simulink model "simu_hapstik_1"  (Simulink 7.7)
settings: Solver=ode45  StartTime=0.0  StopTime=25  RelTol=1e-3
settings Model: Creator=André Frank  LastModifiedBy=André Frank

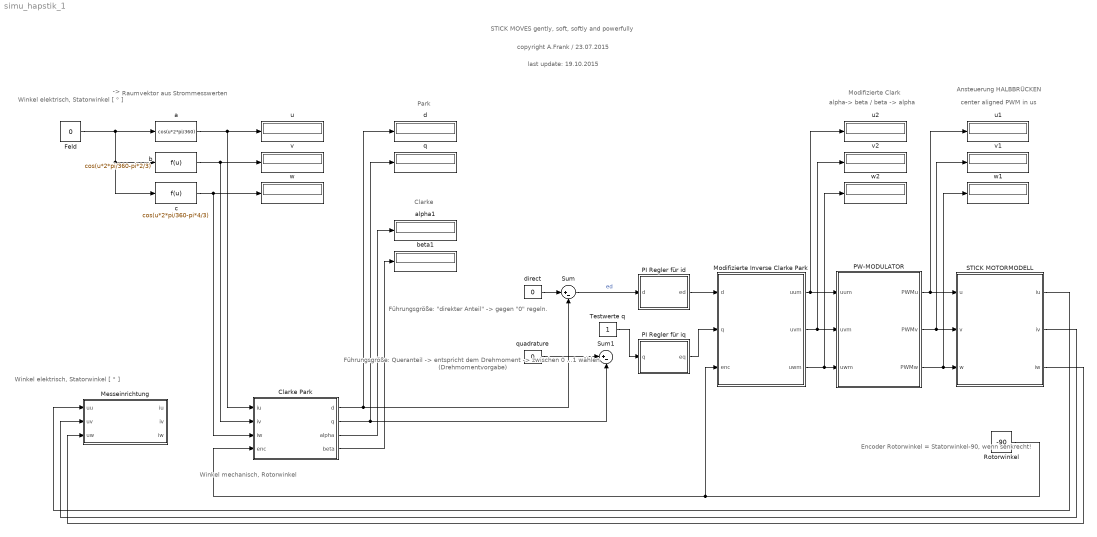
== system simu_hapstik_1 ==
  note: Winkel elektrisch,
      | Statorwinkel
      | [ ° ]
  note: ->
  note: Raumvektor
      | aus Strommesswerten
  note: Encoder
      | Rotorwinkel
      | = Statorwinkel-90,
      | wenn senkrecht!
  note: Führungsgröße:
      | "direkter Anteil"
      | -> gegen "0"
      | regeln.
  note: Führungsgröße:
      | Queranteil
      | -> entspricht dem Drehmoment
      | -> zwischen 0 ...1 wählen
      | (Drehmomentvorgabe)
  note: STICK MOVES
      | gently, soft, softly and powerfully
  note: Clarke
  note: Park
  note: Ansteuerung HALBBRÜCKEN
  note: center aligned PWM
      | in us
  note: Modifizierte Clark
  note: alpha-> beta / beta -> alpha
  note: copyright A.Frank / 23.07.2015
  note: Winkel mechanisch,
      | Rotorwinkel
  note: Winkel elektrisch,
      | Statorwinkel
      | [ ° ]
  note: last update: 19.10.2015
  Clarke Park : Stateflow chart  TreatAsAtomicUnit=on
  Feld : Constant  Value=0
  Messeinrichtung : Stateflow chart  TreatAsAtomicUnit=on
  Modifizierte Inverse Clarke Park : Stateflow chart  TreatAsAtomicUnit=on
  PI Regler für id : Stateflow chart  TreatAsAtomicUnit=on
  PI Regler für iq : Stateflow chart  TreatAsAtomicUnit=on
  PW-MODULATOR : Stateflow chart  TreatAsAtomicUnit=on
  Rotorwinkel : Constant  Value=-90
  STICK MOTORMODELL : Stateflow chart  TreatAsAtomicUnit=on
  Sum : Sum  Inputs=|+-
  Sum1 : Sum  Inputs=|+-
  Testwerte q : Constant
  a : Fcn  Expr=cos(u*2*pi/360)
  alpha1 : Display
  b : Fcn  Expr=cos(u*2*pi/360-pi*2/3)
  beta1 : Display
  c : Fcn  Expr=cos(u*2*pi/360-pi*4/3)
  d : Display
  direct : Constant  Value=0
  q : Display
  quadrature : Constant  Value=0
  u : Display
  u1 : Display
  u2 : Display
  v : Display
  v1 : Display
  v2 : Display
  w : Display
  w1 : Display
  w2 : Display
  wires:
  Feld/1 -> a/1, b/1, c/1
  a/1 -> Clarke Park/1(iu), u/1
  b/1 -> Clarke Park/2(iv), v/1
  c/1 -> Clarke Park/3(iw), w/1
  Clarke Park/3(alpha) -> alpha1/1
  Clarke Park/4(beta) -> beta1/1
  Clarke Park/1(d) -> d/1, Sum/2
  Clarke Park/2(q) -> q/1, Sum1/2
  direct/1 -> Sum/1
  quadrature/1 -> Sum1/1
  Sum/1 -> PI Regler für id/1(d)  "ed"
  PI Regler für iq/1(eq) -> Modifizierte Inverse Clarke Park/2(q)
  PI Regler für id/1(ed) -> Modifizierte Inverse Clarke Park/1(d)
  Modifizierte Inverse Clarke Park/1(uum) -> PW-MODULATOR/1(uum), u2/1
  STICK MOTORMODELL/2(iv) -> Messeinrichtung/2(uv)
  STICK MOTORMODELL/3(iw) -> Messeinrichtung/3(uw)
  PW-MODULATOR/1(PWMu) -> STICK MOTORMODELL/1(u), u1/1
  PW-MODULATOR/2(PWMv) -> STICK MOTORMODELL/2(v), v1/1
  Modifizierte Inverse Clarke Park/2(uvm) -> PW-MODULATOR/2(uvm), v2/1
  Modifizierte Inverse Clarke Park/3(uwm) -> PW-MODULATOR/3(uwm), w2/1
  PW-MODULATOR/3(PWMw) -> STICK MOTORMODELL/3(w), w1/1
  STICK MOTORMODELL/1(iu) -> Messeinrichtung/1(uu)
  Testwerte q/1 -> PI Regler für iq/1(q)
  Rotorwinkel/1 -> Clarke Park/4(enc), Modifizierte Inverse Clarke Park/3(enc)

== matlab function PI Regler für iq ==
  data: q input double; eq output double
function eq = piq (q)


%PI-Regler für die q-Komponente

eq = q;

== matlab function PI Regler für id ==
  data: d input double; ed output double
function ed = pid (d)


%PI-Regler für die d-Komponente

ed = -d;

== matlab function Modifizierte Inverse Clarke Park ==
  data: d input double; q input double; uum output double; uvm output double; uwm output double; enc input double
function [uum,uvm,uwm] = m_inv_clarke_park(d,q,enc)


%{
Modifizierte inverse Clarke Park Transformation
->
Dazu werden in der inversen Clarke-Transformation alpha und beta
getauscht, so dass die beteiligten Vektoren u, v, w die direkten 
Wichtungsanteile der beiden Basisvektoren beinhalten.
Zusätzliche Rechnungen entfallen damit!



- der winkel wird von einem encoder abgenommen
- bei einem encoder mit 200 Schritten sind das 800 Flanken
- 360°/800 Flanken macht eintspricht einer Winkelauflösung von
  0,45°e winkel von grad nach rad wandeln
- bei einem BLDC mit der Struktur 12N14P ist der Winkel zwischen
  benachbarten Raumzeigern 360/(12*14)=2,14°
- nach diesem Winkel liefern die Halls eine neue Kombination

->
- die Auflösung mit dem Encoder ist ca. 4,8x besser!

- Winkel des Encoders von Grad -> Bogenmaß
%}



%{
Hier nur als Hilfsmittel, um nicht bei Änderung vom Statorwinkel den
Rotorwinkel immer mit ändern zu müssen:
enc_b = (enc - 90)* 2*pi/360;
Umrouten im Schaltbild erforderlich!
%}

enc_b = (enc)* 2*pi/360;



%{
inverse Park Transformation: 
2-achs rotorfestes Koordinatensystem ->
2-achs statorfestes Koordinatensystem
%}

alpha = cos(enc_b)* d - sin(enc_b)* q;
beta  = sin(enc_b)* d + cos(enc_b)* q;




%{
inverse Clarke Transformation: 
2-achs statorfestes Koordinatensystem ->
3-achs Koordinatensysten
%}

%{
Original:
uu = alpha
uv = 1/2* (sqrt(3)* beta - alpha);
uw = (-1)* 1/2* (alpha +  sqrt(3)* beta);

Modifiziert:
%}

uum = beta
uvm = 1/2* (sqrt(3)* alpha - beta);
uwm = (-1)* 1/2* (beta +  sqrt(3)* alpha);

== matlab function Clarke Park ==
  data: iu input double; d output double; iv input double; iw input double; enc input double; q output double; alpha output double; beta output double
function [d,q,alpha,beta] = clarke_park(iu,iv,iw,enc)

%{
Clarke Transformation: 
3-achs Koordinatensysten -> 2-achs Koordinatensystem


Hier mit Absicht die volle Berechnung, also ohne Vereinfachungen, 
durchgeführt. 
Stimmt jetzt mit dem Excel-Formeln überein.
%}
 
alpha = 2/3 * (iu - iv/2           - iw/2);
beta  = 2/3 * (sqrt(3)/2 * iv - sqrt(3)/2 * iw);

%{
- der winkel wird von einem encoder abgenommen
- bei einem encoder mit 200 Schritten sind das 800 Flanken
- 360°/800 Flanken macht eintspricht einer Winkelauflösung von
  0,45°e winkel von grad nach rad wandeln
- bei einem BLDC mit der Struktur 12N14P ist der Winkel zwischen
  benachbarten Raumzeigern 360/(12*14)=2,14°
- nach diesem Winkel liefern die Halls eine neue Kombination

->
- die Auflösung mit dem Encoder ist ca. 4,8x besser!
%}


%{
Hier nur als Hilfsmittel, um nicht bei Änderung vom Statorwinkel den
Rotorwinkel immer mit ändern zu müssen:
enc_b = (enc - 90)* 2*pi/360;
Umrouten im Schaltbild erforderlich!
%}

enc_b = (enc)* 2*pi/360;


%{
Park Transformation: 
2-achs statorfestes Koordinatensystem -> 2-achs rotorfestes 
Koordinatensystem
%}

d = cos(enc_b)* alpha + sin(enc_b)* beta;
q = cos(enc_b)* beta  - sin(enc_b)* alpha

== matlab function STICK MOTORMODELL ==
  data: u input double; v input double; w input double; iu output double; iv output double; iw output double
function [iu,iv,iw] = Motormodell(u,v,w)

%{
inverse Clarke Park Transformation: 
3-achs Koordinatensysten -> 2-achs Koordinatensystem
%}


iu=u
iv=v
iw=w

%{
- der winkel wird von einem encoder abgenommen
- bei einem encoder mit 200 Schritten sind das 800 Flanken
- 360°/800 Flanken macht eintspricht einer Winkelauflösung von
  0,45°e winkel von grad nach rad wandeln
- bei einem BLDC mit der Struktur 12N14P ist der Winkel zwischen
  benachbarten Raumzeigern 360/(12*14)=2,14°
- nach diesem Winkel liefern die Halls eine neue Kombination

->
- die Auflösung mit dem Encoder ist ca. 4,8x besser!
%}



%{
Park Transformation: 
2-achs statorfestes Koordinatensystem -> 2-achs rotorfestes 
Koordinatensystem
%}

== matlab function Messeinrichtung ==
  data: iu output double; iv output double; iw output double; uu input double; uv input double; uw input double
function [iu,iv,iw] = Messverstaerker(uu,uv,uw)

%{
inverse Clarke Park Transformation: 
3-achs Koordinatensysten -> 2-achs Koordinatensystem
%}


iu=10*uu
iv=10*uv
iw=10*uw

%{
- der winkel wird von einem encoder abgenommen
- bei einem encoder mit 200 Schritten sind das 800 Flanken
- 360°/800 Flanken macht eintspricht einer Winkelauflösung von
  0,45°e winkel von grad nach rad wandeln
- bei einem BLDC mit der Struktur 12N14P ist der Winkel zwischen
  benachbarten Raumzeigern 360/(12*14)=2,14°
- nach diesem Winkel liefern die Halls eine neue Kombination

->
- die Auflösung mit dem Encoder ist ca. 4,8x besser!
%}



%{
Park Transformation: 
2-achs statorfestes Koordinatensystem -> 2-achs rotorfestes 
Koordinatensystem
%}

== matlab function PW-MODULATOR ==
  data: uum input double; PWMu output double; uvm input double; uwm input double; PWMv output double; PWMw output double
function [PWMu,PWMv,PWMw] = SVPWM(uum,uvm,uwm)
%{

- SVPWM

- uum   -> "Spannung u modifiziert"


- A.Frank 
- 23.07.2015
- 19.10.2015

%}


PWM=100;


% (0,1,1) 0-60 degrees
if uum >= 0
    if uvm >= 0         

        T1s = uvm;
        T2s = uum;
        
        
        %CalcTimes();
        T1 = PWM*T1s;
        T2 = PWM*T2s;
        Tc = (PWM-T1-T2)/2;
        Tb = Tc + T1;
        Ta = Tb + T2;
    
        
        PWMu = Ta;
        PWMv = Tb;
        PWMw = Tc;
    else
        % (1,0,1) 120-180 degrees    
        if uwm >= 0    
            T1s = uum;
            T2s = uwm;
            
            
            %CalcTimes();
            T1 = PWM*T1s;
            T2 = PWM*T2s
            Tc = (PWM-T1-T2)/2;
            Tb = Tc + T1;
            Ta = Tb + T2;
    
            
            PWMu = Tc;
            PWMv = Ta;
            PWMw = Tb;
        else
        % (0,0,1) 60-120 degrees    
            T1s = -uvm;
            T2s = -uwm;
            
            
            %CalcTimes();
            T1 = PWM*T1s;
            T2 = PWM*T2s;
            Tc = (PWM-T1-T2)/2;
            Tb = Tc + T1;
            Ta = Tb + T2;
    
            
            PWMu = Tb;
            PWMv = Ta;
            PWMw = Tc;
        end 
    end
else
   
    if uvm >= 0
        % (1,1,0) 240-300 degrees
        if uwm >= 0    
            T1s = uwm;
            T2s = uvm;
            
            
            %CalcTimes();
            T1 = PWM*T1s;
            T2 = PWM*T2s;
            Tc = (PWM-T1-T2)/2;
            Tb = Tc + T1;
            Ta = Tb + T2;
    
            
            PWMu = Tb;
            PWMv = Tc;
            PWMw = Ta;
        else
        % (0,1,0) 300-0 degrees   
            T1s = -uwm;
            T2s = -uum;
            %CalcTimes();
            T1 = PWM*T1s;
            T2 = PWM*T2s;
            Tc = (PWM-T1-T2)/2;
            Tb = Tc + T1;
            Ta = Tb + T2;
    
            PWMu = Ta;
            PWMv = Tc;
            PWMw = Tb;
        end 
    else
    % (1,0,0) 180-240 degrees   
        T1s = -uum;
        T2s = -uvm;
        
        
        %CalcTimes();
        T1 = PWM*T1s;
        T2 = PWM*T2s;
        Tc = (PWM-T1-T2)/2;
        Tb = Tc + T1;
        Ta = Tb + T2;
   
        
        PWMu = Tc;
        PWMv = Tb;
        PWMw = Ta;  
    end
end
